simulink model "PTB_ConventionalModel"  (R2018a)
settings: Solver=ode23t  StartTime=0.0  StopTime=TimeUS06  RelTol=1e-3
model workspace (MAT data in the model file):
  Af = 4
  Cd = 0.3
  D = 0.322411602927
  DownShiftSpeeds = [11.05  11.05  11.05  11.05  11.05  11.05  11.05  11.05  11.05  11.05  11.05  11.05  19.55  25.5  31.45  35.7  35.7; 18.7  18.7  18.7  18.7  19.125  20.48636  21.33636  23.375  27.28636  30.26136  33.827365  38.76136  46.072635  56.1  64.6  73.1  73.1; 28.9  28.9  28.9  28.9  28.9  30.51364  34.51136  41.56364  47.68636  53.377365  58.477365  65.622635  73.525  81.26136  88.48636  115.6  115.6; 38.675  38.675  38.675  38.675  39.43864  42.41364  47.68636  56.43864  65.11136  72.927365  80.497635  90.01364  100.81136  110.672635  122.4  153  153; 51.425  51.425  51.425  51.425  51.76364  55.077365  62.38864  72.422635  83.3  102  136  425  425  425  425  425  425]
  DrCycles.C505 = [0 1 2 3 4 5 6 7 8 9 10 11 ... (1012 elements, 506x2)]
  DrCycles.FTP = [0 1 2 3 4 5 6 7 8 9 10 11 ... (4956 elements, 2478x2)]
  DrCycles.UDDS = [0 1 2 3 4 5 6 7 8 9 10 11 ... (2746 elements, 1373x2)]
  DrCycles.HWFET = [0 1 2 3 4 5 6 7 8 9 10 11 ... (1532 elements, 766x2)]
  DrCycles.US06 = [0 1 2 3 4 5 6 7 8 9 10 11 ... (1194 elements, 597x2)]
  DrCycles.US06City = [0 1 2 3 4 5 6 7 8 9 10 11 ... (466 elements, 233x2)]
  DrCycles.US06Hwy = [0 1 2 3 4 5 6 7 8 9 10 11 ... (742 elements, 371x2)]
  I = 0.25
  Kbr = 10000
  P = 15
  PedalPositions = [0 6.2485 12.4969 18.7454 24.9939 31.2424 37.4908 43.7393 49.9878 56.2363 62.4847 68.7332 74.9817 81.2302 87.4786 93.7271 99.9756]
  TimeHWFET = 765
  TimeUDDS = 1372
  TimeUS06 = 596
  UpShiftSpeeds = [12.75  12.75  12.75  12.75  12.75  12.75  15.552365  17.08636  18.7  20.227365  23.46136  27.625  31.702365  36.63636  42.5  42.5  42.5; 20.997635  20.997635  20.997635  20.997635  21.927365  24.902365  28.727365  31.78864  35.275  39.697635  46.41136  51.85  59.672635  67.48864  78.2  78.2  78.2; 31.45  31.45  31.45  31.45  34.172635  41.052365  47.175  52.952365  59.5  68  76.5  85  93.5  106.25  119.85  119.85  119.85; 42.16136  42.16136  42.16136  43.947635  47.002365  54.31364  63.325  71.227365  79.222635  88.06136  98.852365  109.052365  118.402365  128.86136  157.25  157.25  157.25; 55.58864  55.58864  55.58864  58.052365  61.53864  72.077365  85.51136  96.81364  255  255  255  255  255  255  255  255  255]
  axle_b = 10
  axle_k = 5000
  convAxle_wc = 500
  diffRatio = 3.4
  driveshaft_b = 10
  driveshaft_k = 2500
  driveshaft_wc = 500
  engineSpeedPoints_rpm = [750 1053.57142857 1357.14285714 1660.71428571 1964.28571429 2267.85714286 2571.42857143 2875 3178.57142857 3482.14285714 3785.71428571 4089.28571429 4392.85714286 4696.42857143 5000]
  engineTorqueMap_Nm = [-13.6738264269 15.0034460821 26.4289521305 37.8539339756 49.2854604964 60.7146317399 72.0173711595 77.7345012802 77.7345012802 77.7345012802 77.7345012802 77.7345012802 ... (240 elements, 16x15)]
  engineTorquePoints_Nm = [0 15 26.4285714286 37.8571428571 49.2857142857 60.7142857143 72.1428571429 83.5714285714 95 106.428571429 117.857142857 129.285714286 140.714285714 152.142857143 163.571428571 175]
  vehicleMass = 1500
  wheelRadius = 0.35
libraries: Wheels_Driver_VehDyn_Lib x3, autolibsharedcoupling x2, simulink x2, autolibshareddiff x1, autolibsharedtransfixedgear x1, autolibenginesystems x1
(part 1 of 3)
settings Model: Creator=emarquez  LastModifiedBy=emarquez
settings DebuggingCC: AlgebraicLoopMsg=none
settings CodeAppCC: StateflowObjectComments=on
settings SimscapeCC: SimscapeNormalizeSystem=off

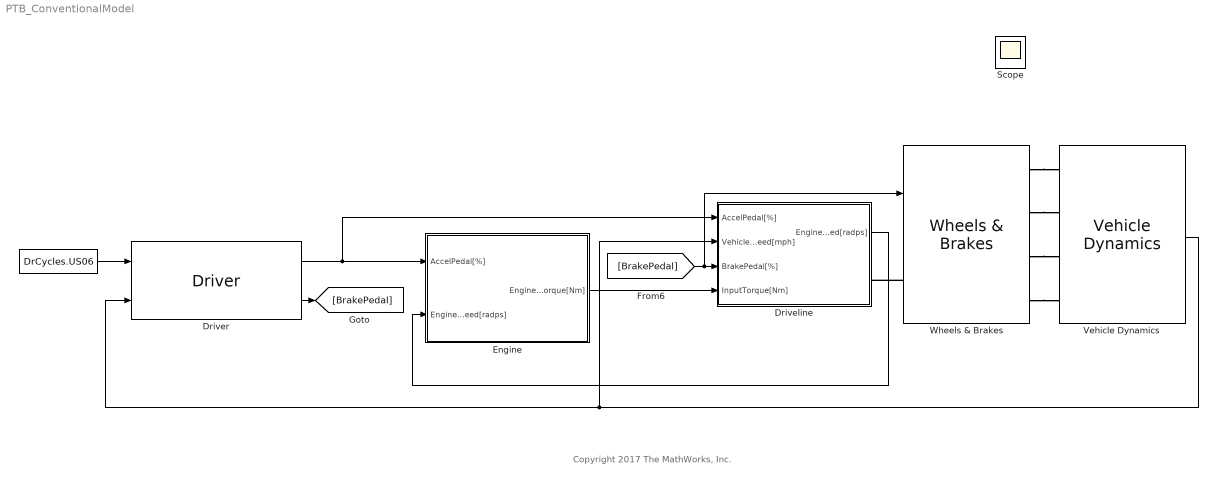
== system PTB_ConventionalModel ==
  note: Copyright 2017 The MathWorks, Inc.
  " " : FromWorkspace  Tag=DriveCycle  VariableName=DrCycles.US06  SampleTime=0
  Driveline : Subsystem
  Driver : Wheels_Driver_VehDyn_Lib/Driver
  Engine : Subsystem
  Vehicle Dynamics : Wheels_Driver_VehDyn_Lib/Vehicle Dynamics
  Wheels & Brakes : Wheels_Driver_VehDyn_Lib/Wheels & Brakes
  Scope : Scope
  wires:
  [BrakePedal] -> Wheels & Brakes/1, Driveline/3(BrakePedal[%])
  Vehicle Dynamics/1 -> Driver/2, Driveline/2(VehicleSpeed[mph])
  Driver/1 -> Driveline/1(AccelPedal[%]), Engine/1(AccelPedal[%])
  Driver/2 -> [BrakePedal]
  " "/1 -> Driver/1
  Engine/1(EngineTorque[Nm]) -> Driveline/4(InputTorque[Nm])
  Driveline/1(EngineSpeed[radps]) -> Engine/2(EngineSpeed[radps])
  connections:
  Wheels & Brakes/LConn1 -- Driveline/RConn1
  Wheels & Brakes/RConn1 -- Vehicle Dynamics/LConn1
  Wheels & Brakes/RConn2 -- Vehicle Dynamics/LConn2
  Wheels & Brakes/RConn3 -- Vehicle Dynamics/LConn3
  Wheels & Brakes/RConn4 -- Vehicle Dynamics/LConn4

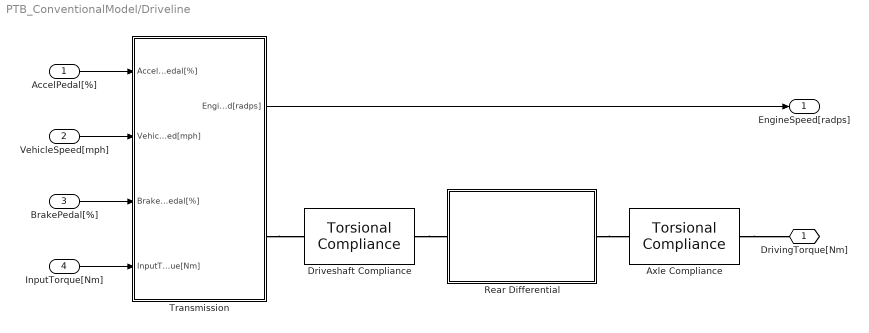
== system PTB_ConventionalModel/Driveline ==
  AccelPedal[%] : Inport
  VehicleSpeed[mph] : Inport  Port=2
  BrakePedal[%] : Inport  Port=3
  InputTorque[Nm] : Inport  Port=4
  Axle Compliance : autolibsharedcoupling/Torsional Compliance  port_config=Two-way connection  k=axle_k  b=axle_b  theta_o=0  domega_o=0  omega_c=convAxle_wc  blkID=0  aMode=1
      settings: SourceProductName=Powertrain Blockset  SourceProductBaseCode=PW
  Driveshaft Compliance : autolibsharedcoupling/Torsional Compliance  port_config=Two-way connection  k=driveshaft_k  b=driveshaft_b  theta_o=0  domega_o=0  omega_c=driveshaft_wc  blkID=0
      settings: SourceProductName=Powertrain Blockset  SourceProductBaseCode=PW
  Rear Differential : Subsystem
  Transmission : Subsystem
  DrivingTorque[Nm] : PMIOPort  Side=Right
  EngineSpeed[radps] : Outport
  wires:
  Transmission/1(EngineSpeed[radps]) -> EngineSpeed[radps]/1
  InputTorque[Nm]/1 -> Transmission/4(InputTorque[Nm])
  AccelPedal[%]/1 -> Transmission/1(AccelPedal[%])
  VehicleSpeed[mph]/1 -> Transmission/2(VehicleSpeed[mph])
  BrakePedal[%]/1 -> Transmission/3(BrakePedal[%])
  connections:
  Axle Compliance/RConn1 -- DrivingTorque[Nm]/RConn1
  Rear Differential/RConn1 -- Axle Compliance/LConn1
  Driveshaft Compliance/RConn1 -- Rear Differential/LConn1
  Transmission/RConn1 -- Driveshaft Compliance/LConn1
